simulink model "Real_system_controller"  (R2015a)
settings: Solver=ode45  StartTime=0.0  StopTime=10.0  RelTol=1e-3
values from neighbouring files (symbols this model uses):
  Nbar = inv(C*inv(eye(size(A))-A+B*K)*B)    [Controller_Design.m]    (also in Controller_Design_Real.m)
undefined symbols (not defined in the file or in its folder): A, B, C, D, K, M, MIO, National_Instruments, PCI
libraries: sldrtlib x3
settings Model: Creator=alunos  LastModifiedBy=alunos
settings DataIOCC: LimitDataPoints=off

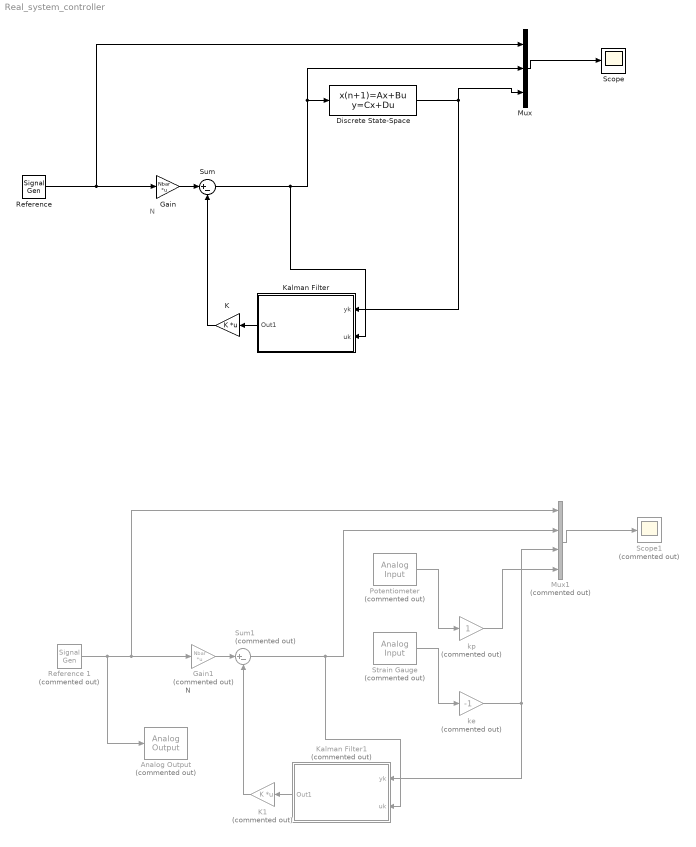
== system Real_system_controller ==
  note: N
  note: N
  " Potentiometer" : sldrtlib/Analog Input  Commented=on  SampleTime=0.01  MaxMissedTicks=10  ShowMissedTicks=off  YieldWhenWaiting=off  DrvName=National_Instruments/PCI-MIO-16E-4  DrvAddress=4294967295  DrvOptions=[0 0 0 0 0 0]  Channels=1  RangeMode=1  VoltRange=1  DataType=1
      settings: AttributesFormatString=National Instruments\nPCI-MIO-16E-4 [auto]
  Analog Output : sldrtlib/Analog Output  Commented=on  SampleTime=0.01  MaxMissedTicks=10  ShowMissedTicks=off  YieldWhenWaiting=off  DrvName=National_Instruments/PCI-MIO-16E-4  DrvAddress=4294967295  DrvOptions=[0 0 0 0 0 0]  Channels=1  RangeMode=1  VoltRange=1  InitialValue=0  FinalValue=0
      settings: AttributesFormatString=National Instruments\nPCI-MIO-16E-4 [auto]
  Discrete State-Space : DiscreteStateSpace  A=A  B=B  C=C  D=D  SampleTime=0.02
  Gain : Gain  Gain=Nbar  Multiplication=Matrix(K*u)
  Gain1 : Gain  Commented=on  Gain=Nbar  Multiplication=Matrix(K*u)
  K : Gain  Gain=K  Multiplication=Matrix(K*u)
  K1 : Gain  Commented=on  Gain=K  Multiplication=Matrix(K*u)
  Kalman Filter : Subsystem
  Kalman Filter1 : Subsystem  Commented=on
  Mux : Mux  Inputs=3
  Mux1 : Mux  Commented=on
  "Reference " : SignalGenerator  WaveForm=square  Amplitude=25  Frequency=0.4
  Reference 1 : SignalGenerator  Commented=on  WaveForm=square  Amplitude=25  Frequency=0.4
  Scope : Scope
      settings: ShowLegends=on
  Scope1 : Scope  Commented=on
      settings: ShowLegends=on
  "Strain Gauge " : sldrtlib/Analog Input  Commented=on  SampleTime=0.01  MaxMissedTicks=10  ShowMissedTicks=off  YieldWhenWaiting=off  DrvName=National_Instruments/PCI-MIO-16E-4  DrvAddress=4294967295  DrvOptions=[0 0 0 0 0 0]  Channels=2  RangeMode=1  VoltRange=1  DataType=1
      settings: AttributesFormatString=National Instruments\nPCI-MIO-16E-4 [auto]
  Sum : Sum  Inputs=|+-
  Sum1 : Sum  Commented=on  Inputs=|+-
  "ke " : Gain  Commented=on  Gain=-1
  "kp " : Gain  Commented=on
  wires:
  Reference 1/1 -> Analog Output/1, Mux1/1, Gain1/1
  Gain1/1 -> Sum1/1
  Kalman Filter1/1(Out1) -> K1/1
  Sum1/1 -> Kalman Filter1/2("uk "), Mux1/2
  K1/1 -> Sum1/2
  Mux1/1 -> Scope1/1
  "Strain Gauge "/1 -> "ke "/1
  " Potentiometer"/1 -> "kp "/1
  "ke "/1 -> Mux1/3, Kalman Filter1/1("yk ")
  "kp "/1 -> Mux1/4
  "Reference "/1 -> Mux/1, Gain/1
  Gain/1 -> Sum/1
  Kalman Filter/1(Out1) -> K/1
  Sum/1 -> Kalman Filter/2("uk "), Mux/2, Discrete State-Space/1
  K/1 -> Sum/2
  Mux/1 -> Scope/1
  Discrete State-Space/1 -> Mux/3, Kalman Filter/1("yk ")

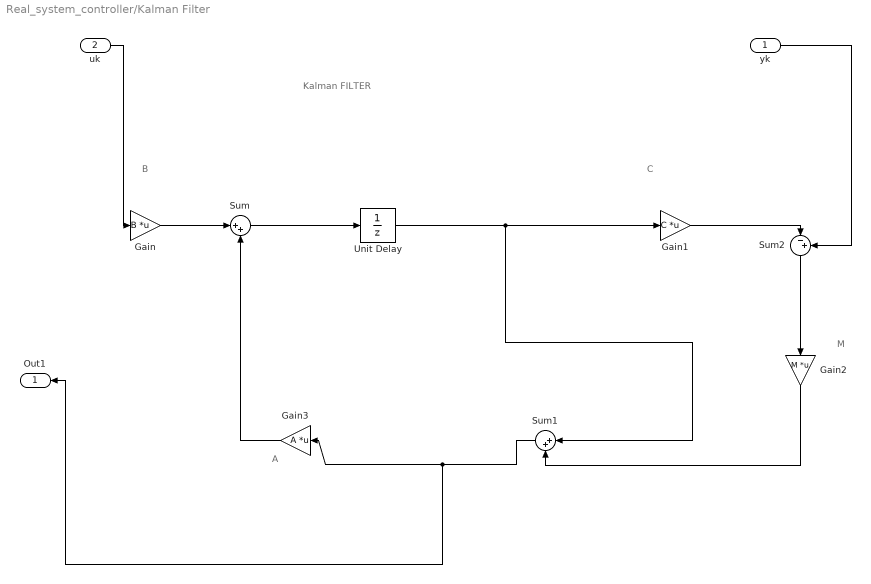
== system Real_system_controller/Kalman Filter ==
  note: Kalman FILTER
  note: M
  note: C
  note: B
  note: A
  "yk " : Inport
  "uk " : Inport  Port=2
  Gain : Gain  Gain=B  Multiplication=Matrix(K*u)
  Gain1 : Gain  Gain=C  Multiplication=Matrix(K*u)
  Gain2 : Gain  Gain=M  Multiplication=Matrix(K*u)
  Gain3 : Gain  Gain=A  Multiplication=Matrix(K*u)
  Sum : Sum  Inputs=|++
  Sum1 : Sum  Inputs=|++
  Sum2 : Sum  Inputs=|-+
  Unit Delay : UnitDelay  SampleTime=-1
  Out1 : Outport
  wires:
  Gain1/1 -> Sum2/1
  Gain2/1 -> Sum1/2
  "yk "/1 -> Sum2/2
  Unit Delay/1 -> Sum1/1, Gain1/1
  Gain/1 -> Sum/1
  Sum/1 -> Unit Delay/1
  Gain3/1 -> Sum/2
  "uk "/1 -> Gain/1
  Sum2/1 -> Gain2/1
  Sum1/1 -> Out1/1, Gain3/1

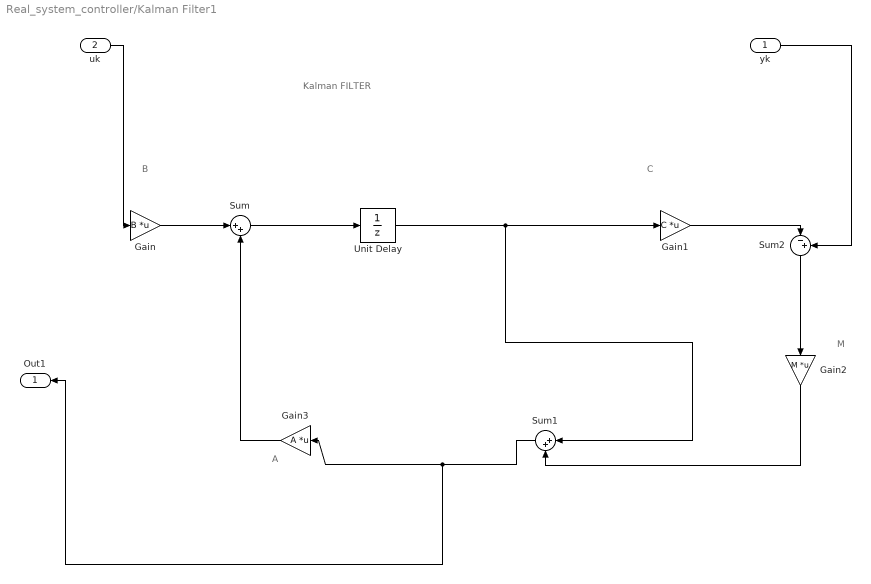
== system Real_system_controller/Kalman Filter1 ==
  note: Kalman FILTER
  note: M
  note: C
  note: B
  note: A
  "yk " : Inport
  "uk " : Inport  Port=2
  Gain : Gain  Gain=B  Multiplication=Matrix(K*u)
  Gain1 : Gain  Gain=C  Multiplication=Matrix(K*u)
  Gain2 : Gain  Gain=M  Multiplication=Matrix(K*u)
  Gain3 : Gain  Gain=A  Multiplication=Matrix(K*u)
  Sum : Sum  Inputs=|++
  Sum1 : Sum  Inputs=|++
  Sum2 : Sum  Inputs=|-+
  Unit Delay : UnitDelay  SampleTime=-1
  Out1 : Outport
  wires:
  Gain1/1 -> Sum2/1
  Gain2/1 -> Sum1/2
  "yk "/1 -> Sum2/2
  Unit Delay/1 -> Sum1/1, Gain1/1
  Gain/1 -> Sum/1
  Sum/1 -> Unit Delay/1
  Gain3/1 -> Sum/2
  "uk "/1 -> Gain/1
  Sum2/1 -> Gain2/1
  Sum1/1 -> Out1/1, Gain3/1
